simulink model "untitled"  (R2024a)
settings: Solver=FixedStepDiscrete  StartTime=0.0  StopTime=50  FixedStep=0.01  RelTol=1e-3
settings Model: Creator=Windy  LastModifiedBy=Windy

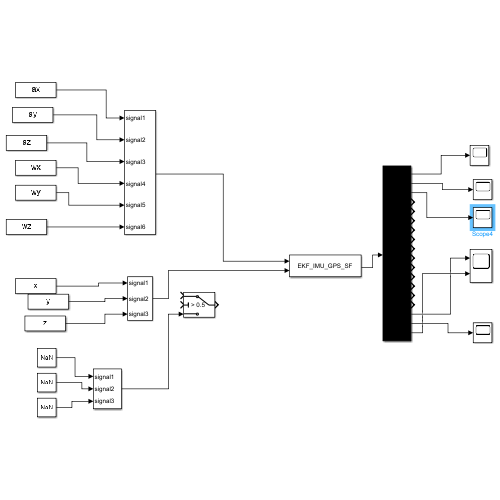
[thumbnail: Simulink's stored preview of the top-level diagram]
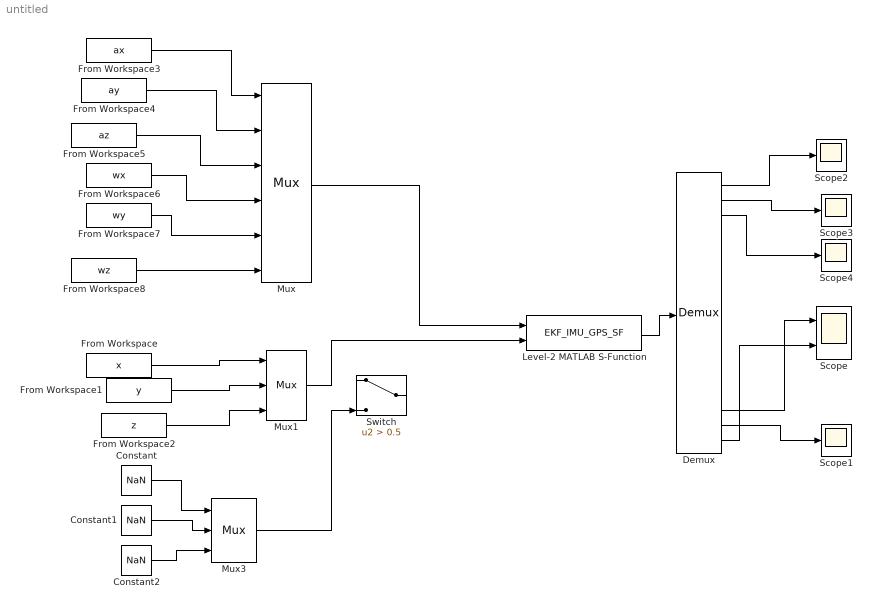
== system untitled ==
  Constant : Constant  Value=NaN
  Constant1 : Constant  Value=NaN
  Constant2 : Constant  Value=NaN
  Demux : Demux  Outputs=18
  From Workspace : FromWorkspace  VariableName=x
  From Workspace1 : FromWorkspace  VariableName=y
  From Workspace2 : FromWorkspace  VariableName=z
  From Workspace3 : FromWorkspace  VariableName=ax
  From Workspace4 : FromWorkspace  VariableName=ay
  From Workspace5 : FromWorkspace  VariableName=az
  From Workspace6 : FromWorkspace  VariableName=wx
  From Workspace7 : FromWorkspace  VariableName=wy
  From Workspace8 : FromWorkspace  VariableName=wz
  Level-2 MATLAB S-Function : M-S-Function  FunctionName=EKF_IMU_GPS_SF  Parameters=9
  Mux : Mux  Inputs=6
      settings: DisplayOption=signals
  Mux1 : Mux  Inputs=3
      settings: DisplayOption=signals
  Mux3 : Mux  Inputs=3
      settings: DisplayOption=signals
  Scope : Scope  NumInputPorts=2
  Scope{1..4} (4 alike) : Scope
  Switch : Switch  Criteria=u2 > Threshold  Threshold=0.5  SaturateOnIntegerOverflow=off  InputSameDT=off
  wires:
  Level-2 MATLAB S-Function/1 -> Demux/1
  Demux/16 -> Scope/1
  Demux/18 -> Scope/2
  Demux/17 -> Scope1/1
  From Workspace3/1 -> Mux/1
  From Workspace4/1 -> Mux/2
  From Workspace5/1 -> Mux/3
  From Workspace6/1 -> Mux/4
  From Workspace7/1 -> Mux/5
  From Workspace8/1 -> Mux/6
  From Workspace2/1 -> Mux1/3
  From Workspace1/1 -> Mux1/2
  From Workspace/1 -> Mux1/1
  Constant/1 -> Mux3/1
  Constant1/1 -> Mux3/2
  Constant2/1 -> Mux3/3
  Mux3/1 -> Switch/3
  Mux/1 -> Level-2 MATLAB S-Function/1
  Mux1/1 -> Level-2 MATLAB S-Function/2
  Demux/1 -> Scope2/1
  Demux/2 -> Scope3/1
  Demux/3 -> Scope4/1
